simulink model "perfect_tone_iq"  (R2014b)
settings: Solver=ode45  StartTime=0.0  StopTime=inf  RelTol=1e-3
settings Model: Creator=Ben  LastModifiedBy=Ben

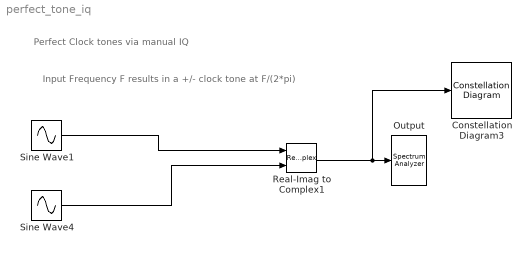
== system perfect_tone_iq ==
  note: Input Frequency F results in a +/- clock tone at F/(2*pi)
  note: Perfect Clock tones via manual IQ
  Constellation Diagram3 : ConstellationDiagram
  Output : SpectrumAnalyzer
  Real-Imag to Complex1 : RealImagToComplex
  Sine Wave1 : Sin  Frequency=10*2*3.14*1000  Phase=-pi/2  SampleTime=1/128000
  Sine Wave4 : Sin  Frequency=10*2*3.14*1000  SampleTime=1/128000
  wires:
  Sine Wave1/1 -> Real-Imag to Complex1/1
  Sine Wave4/1 -> Real-Imag to Complex1/2
  Real-Imag to Complex1/1 -> Constellation Diagram3/1, Output/1
